simulink model "Example_of_simple_controls_to_XPlane"  (R2021b)
settings: Solver=VariableStepAuto  StartTime=0.0  StopTime=Inf  RelTol=1e-3
libraries: arduinolib x1, svdutilitieslib x1, sldrtlib x1, dspnetwork x1
settings Model: Creator=setup  LastModifiedBy=dmgp1
settings DataIOCC: SaveState=on

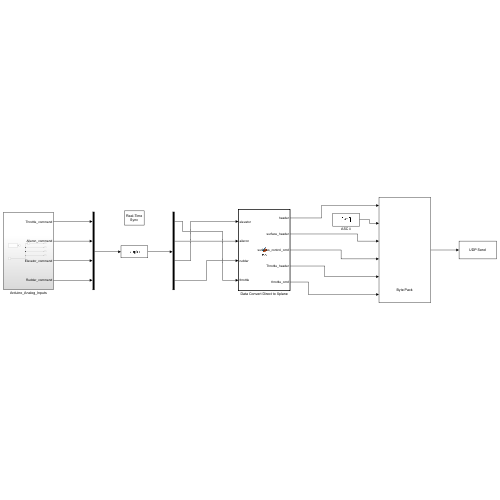
[thumbnail: Simulink's stored preview of the top-level diagram]
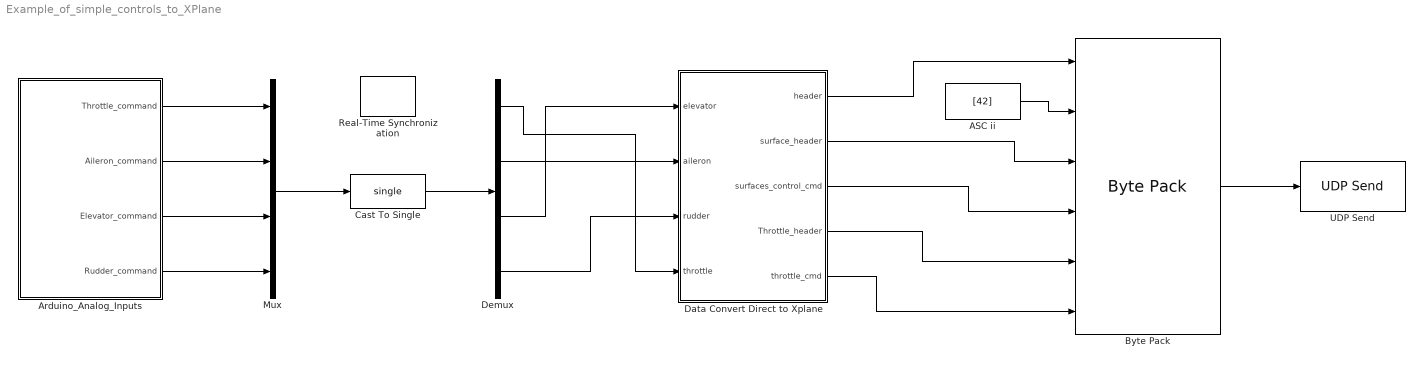
== system Example_of_simple_controls_to_XPlane ==
  ASC ii : Constant  Value=[42]  OutDataTypeStr=uint8
  Arduino_Analog_Inputs : Subsystem
  Byte Pack : svdutilitieslib/Byte Pack  maskPackedDataType=uint8  datatypes={'uint8','uint8','uint8','single','uint8','single'}  byteAlign=1  blockPlatform=arduinoert
      settings: SourceProductBaseCode=ANDROID,ARDUINO,ML_ARDUINO,ECCORTEXA,ECCORTEXR,SC_BEAGLEBONE_BLUE,EC_FREEDOM_BOARD,EC_FRDM_K64F,INTEL_BLOCKSET,MICROBIT,NUCLEO,NVIDIA,PX4AUTOPILOTS,RASPPIIO,STMICRODIS,TIC2000,XILINX_BLOCKSET
  Cast To Single : DataTypeConversion  OutDataTypeStr=single
  Data Convert Direct to Xplane : MATLAB Function  TreatAsAtomicUnit=on
  Demux : Demux
  Mux : Mux
  Real-Time Synchronization : sldrtlib/Real-Time Synchronization  SampleTime=0.02  MaxMissedTicks=20  ShowMissedTicks=off  YieldWhenWaiting=off
  UDP Send : dspnetwork/UDP Send  remoteURL='127.0.0.1'  remotePort=49000  localURL='0.0.0.0'  localPortSource=Automatically determine  localPort=-1  sendBufferSize=8192  sampletime=-1  blockPlatform=[]  separateLengthPort=0
  wires:
  Data Convert Direct to Xplane/1(header) -> Byte Pack/1
  ASC ii/1 -> Byte Pack/2
  Mux/1 -> Cast To Single/1
  Cast To Single/1 -> Demux/1
  Arduino_Analog_Inputs/1(Throttle_command) -> Mux/1
  Arduino_Analog_Inputs/2(Aileron_command) -> Mux/2
  Arduino_Analog_Inputs/3(Elevator_command) -> Mux/3
  Arduino_Analog_Inputs/4(Rudder_command) -> Mux/4
  Demux/1 -> Data Convert Direct to Xplane/4(throttle)
  Demux/2 -> Data Convert Direct to Xplane/2(aileron)
  Demux/3 -> Data Convert Direct to Xplane/1(elevator)
  Demux/4 -> Data Convert Direct to Xplane/3(rudder)
  Data Convert Direct to Xplane/2(surface_header) -> Byte Pack/3
  Data Convert Direct to Xplane/3(surfaces_control_cmd) -> Byte Pack/4
  Data Convert Direct to Xplane/4(Throttle_header) -> Byte Pack/5
  Data Convert Direct to Xplane/5(throttle_cmd) -> Byte Pack/6
  Byte Pack/1 -> UDP Send/1

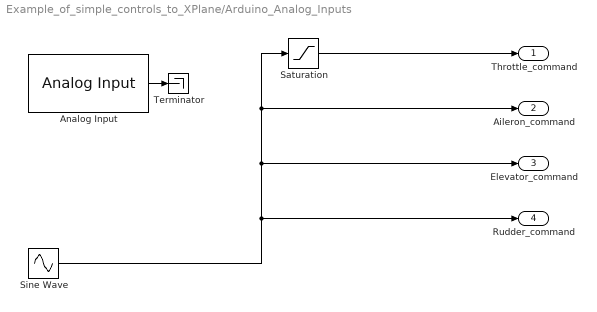
== system Example_of_simple_controls_to_XPlane/Arduino_Analog_Inputs ==
  Analog Input : arduinolib/Analog Input  pinNumber=4  ReadResultsOnly=off  ConversionTriggerSource=Software  ExternalTriggerType=uint32( 0 )  OutputDataType=uint16  EnableConversionCompleteNotify=off  EnableOuputStatus=off  SampleTime=-1  blockPlatform=arduino
  Saturation : Saturate  UpperLimit=1  LowerLimit=0
  Sine Wave : Sin  SampleTime=0
  Terminator : Terminator
  Throttle_command : Outport
  Aileron_command : Outport  Port=2
  Elevator_command : Outport  Port=3
  Rudder_command : Outport  Port=4
  wires:
  Sine Wave/1 -> Aileron_command/1, Saturation/1, Elevator_command/1, Rudder_command/1
  Saturation/1 -> Throttle_command/1
  Analog Input/1 -> Terminator/1

== matlab function Example_of_simple_controls_to_XPlane/Data Convert Direct to Xplane ==
  data: elevator input; aileron input; rudder input; header output; surface_header output; surfaces_control_cmd output; Throttle_header output; throttle_cmd output; throttle input
function [header,surface_header, surfaces_control_cmd,Throttle_header, throttle_cmd] = fcn(elevator, aileron, rudder, throttle) % ,trim_control_cmd // elevator_trim, aileron_trim, rudder_trim,
    header = [uint8(68) uint8(65) uint8(84) uint8(65)]; 

    No_Comand = single(-999);

    surface_header = uint8([uint8(8) uint8(0) uint8(0) uint8(0)]);
    surfaces_control_cmd = [elevator aileron rudder No_Comand No_Comand No_Comand No_Comand No_Comand];

%     Trim_header = typecast(uint8([uint8(13) uint8(0) uint8(0) uint8(0)]), 'single');
%     trim_control_cmd = [ Trim_header elevator_trim aileron_trim rudder_trim No_Comand No_Comand No_Comand No_Comand No_Comand Trim_header No_Comand aileron_trim rudder_trim No_Comand No_Comand No_Comand No_Comand No_Comand];

    Throttle_header = uint8([uint8(25) uint8(0) uint8(0) uint8(0)]);
    throttle_cmd = [throttle No_Comand No_Comand No_Comand No_Comand No_Comand No_Comand No_Comand];

end

% function [header,location_header, location_package] = fcn(X,Y,Altitude) % ,trim_control_cmd // elevator_trim, aileron_trim, rudder_trim,
%     header = [uint8(68) uint8(65) uint8(84) uint8(65)]; 
% 
%     No_Comand = single(-999);
% 
%     location_header = uint8([uint8(21) uint8(0) uint8(0) uint8(0)]);
%     location_package = single([X Altitude Y -42 0 24 No_Comand No_Comand]);
% 
% end

% function [header,location_header, location_package] = fcn(pitch,roll,heading) % ,trim_control_cmd // elevator_trim, aileron_trim, rudder_trim,
%     header = [uint8(68) uint8(65) uint8(84) uint8(65)]; 
% 
%     No_Comand = single(-999);
% 
%     location_header = uint8([uint8(17) uint8(0) uint8(0) uint8(0)]);
%     location_package = single([pitch roll heading No_Comand No_Comand No_Comand No_Comand No_Comand]);
% 
% end

% function [header,speeds_header, speed_package,rotation_header,rotation_package,surface_header, surfaces_package,throttle_header,throttle_package] = fcn(u,v,w,P,Q,R,throttle,aileron,elevator,rudder) % ,trim_control_cmd // elevator_trim, aileron_trim, rudder_trim,
%     header = [uint8(68) uint8(65) uint8(84) uint8(65)]; 
% 
%     No_Comand = single(-999);
% 
%     speeds_header = uint8([uint8(21) uint8(0) uint8(0) uint8(0)]);
%     speed_package = single([No_Comand No_Comand No_Comand u -w v No_Comand No_Comand]);
% 
%     rotation_header = uint8([uint8(17) uint8(0) uint8(0) uint8(0)]);
%     rotation_package = single([Q P No_Comand No_Comand No_Comand No_Comand No_Comand No_Comand]);
% 
%     surface_header = uint8([uint8(8) uint8(0) uint8(0) uint8(0)]);
%     surfaces_package = [elevator aileron rudder No_Comand No_Comand No_Comand No_Comand No_Comand];
% 
%     throttle_header = uint8([uint8(25) uint8(0) uint8(0) uint8(0)]);
%     throttle_package = [throttle No_Comand No_Comand No_Comand No_Comand No_Comand No_Comand No_Comand];
% 
% end
